simulink model "Flyback_Converter_PartA_16a"  (Simulink 8.7)
settings: Solver=ode5  SolverMode=SingleTasking  StartTime=0.0  StopTime=0.005  FixedStep=1e-7  MaxStep=1e-4  RelTol=1e-3
libraries: powerlib x14
settings Model: Creator=WINTER-SOLDIER  LastModifiedBy=nehaj
settings DataIOCC: LimitDataPoints=off  SaveFormat=Dataset
settings DebuggingCC: UnderspecifiedInitializationDetection=Simplified  MergeDetectMultiDrivingBlocksExec=error  SFUnexpectedBacktrackingDiag=error  SFNoUnconditionalDefaultTransitionDiag=error
settings HardwareCC: ProdBitPerPointer=64  ProdLargestAtomicFloat=Float  ProdIntDivRoundTo=Zero  ProdEndianess=LittleEndian  ProdWordSize=64  ProdHWDeviceType=Intel->x86-64 (Windows64)
settings ModelReferenceCC: PropagateSignalLabelsOutOfModel=on
settings GRTTargetCC: TargetLangStandard=C99 (ISO)  GeneratePreprocessorConditionals=Use local settings
settings ConfigComp: CovMetricSettings=dwe  CovHtmlReporting=off  CovSaveCumulativeToWorkspaceVar=off  CovSaveSingleToWorkspaceVar=off  CovModelRefEnable=off  CovExternalEMLEnable=on

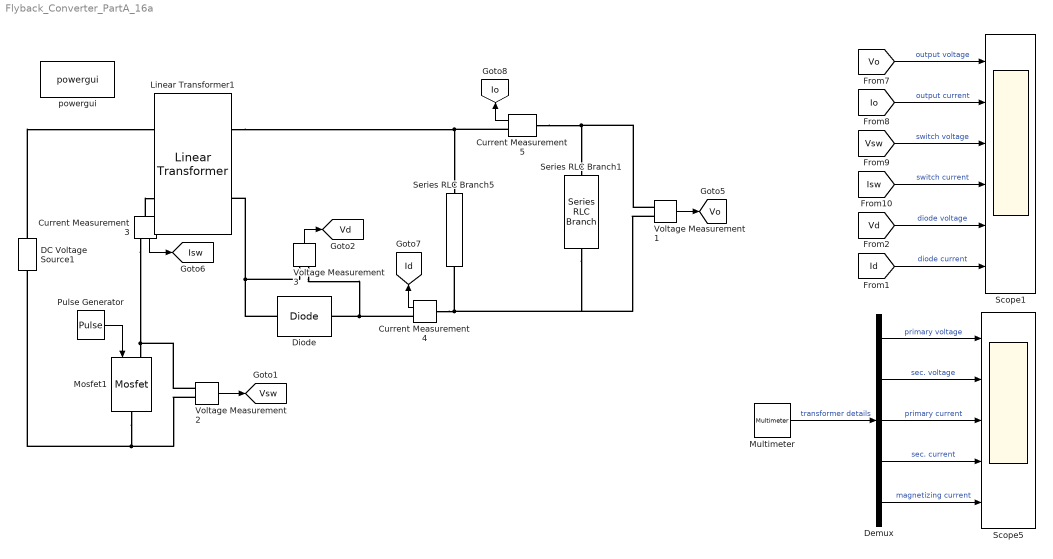
== system Flyback_Converter_PartA_16a ==
  Current Measurement3 : powerlib/Measurements/Current Measurement  PhasorSimulation=off  OutputType=Complex  PSBequivalent=0
  Current Measurement4 : powerlib/Measurements/Current Measurement  PhasorSimulation=off  OutputType=Complex  PSBequivalent=0
  Current Measurement5 : powerlib/Measurements/Current Measurement  PhasorSimulation=off  OutputType=Complex  PSBequivalent=0
  DC Voltage Source1 : powerlib/Electrical Sources/DC Voltage Source  Amplitude=20  Measurements=None
  Demux : Demux  Outputs=5
  Diode : powerlib/Power Electronics/Diode  Ron=1e-6  Lon=0  Vf=0  IC=0  UseSnubber=0  Rs=inf  Cs=0  Measurements=off
  Linear Transformer1 : powerlib/Elements/Linear Transformer  UNITS=SI  NominalPower=[20 100000 ]  winding1=[30 0 0]  winding2=[10 0 0]  ThreeWindings=off  winding3=[3.15e+05 0.7938 0.084225]  RmLm=[inf 250e-6]  Measurements=All voltages and currents  DataType=on
  Mosfet1 : powerlib/Power Electronics/Mosfet  Ron=1e-6  Lon=0  Rd=1e-6  Vfd=0  IC=0  Rs=1e12  Cs=inf  Measurements=off
  Multimeter : powerlib/Measurements/Multimeter  PhasorSimulation=off  OutputType=Complex  sel=[1 2 3 4 6]  L=7  Gain=[1 1 1 1 1]  yselected={'Uw1: Linear Transformer1','Uw2: Linear Transformer1','Iw1: Linear Transformer1','Iw2: Linear Transformer1','Imag: Linear Transformer1'};  PSBOutputType=1  PSBequivalent=0  AxesSetting=[0,0.1,-100,100]  Display=0  SavedBlockNames=-11
  Pulse Generator : DiscretePulseGenerator  PulseType=Time based  Period=1/100000  PulseWidth=50
  Scope1 : Scope  NumInputPorts=6
  Scope5 : Scope  NumInputPorts=5
  Series RLC Branch1 : powerlib/Elements/Series RLC Branch  LConnTagsString=__new0  RConnTagsString=__new0  BranchType=R  Resistance=1.5  Inductance=1e-3  SetiL0=off  InitialCurrent=0  Capacitance=1e-6  Setx0=off  InitialVoltage=0  Measurements=None
  Series RLC Branch5 : powerlib/Elements/Series RLC Branch  LConnTagsString=__new0  RConnTagsString=__new0  BranchType=C  Resistance=0  Inductance=1e-3  SetiL0=off  InitialCurrent=0  Capacitance=100e-6  Setx0=off  InitialVoltage=0  Measurements=None
  Voltage Measurement1 : powerlib/Measurements/Voltage Measurement  PhasorSimulation=off  OutputType=Complex  PSBequivalent=0
  Voltage Measurement2 : powerlib/Measurements/Voltage Measurement  PhasorSimulation=off  OutputType=Complex  PSBequivalent=0
  Voltage Measurement3 : powerlib/Measurements/Voltage Measurement  PhasorSimulation=off  OutputType=Complex  PSBequivalent=0
  powergui : powerlib/powergui  Priority=1  SimulationMode=Discrete  SampleTime=1e-7  frequency=60  Iterations=50  frequencyindice=0  Pbase=100e6  ErrMax=1e-4  UnitsV=kV  UnitsW=MW  buscounter=0  FunctionMessages=off  echomessages=off  EnableUseOfTLC=off  CurrentSourceSwitches=off  DisableSnubberDevices=off  DisableRonSwitches=off  DisableVfSwitches=off  DisplayEquations=off  SolverType=Tustin/Backward Euler (TBE)  Interpol=off  ExternalGateDelay=off  methode=off  Ts=100  x0status=blocks  SPID=on  SwTol=0  HookPort=off  RestoreLinks=warning  ResistiveCurrentMeasurement=off  Frange=[0:2:500]  Ylog=off  Xlog=on  ShowGrid=off  save=off  variable=ZData  structure=0  ZoomFFT=off  StartTime=0.0  cycles=1  DisplayStyle=1  fundamental=60  FreqAxis=off  MaxFrequency=1000  frequencyindicesteady=1  RmsSteady=1  display=off
  tag scope: Id=global, Io=global, Isw=global, Vd=global, Vo=global, Vsw=global
  wires:
  Voltage Measurement1/1 -> [Vo]
  Pulse Generator/1 -> Mosfet1/1
  Current Measurement5/1 -> [Io]
  Current Measurement3/1 -> [Isw]
  Current Measurement4/1 -> [Id]
  [Vsw] -> Scope1/3  "switch voltage"
  [Vo] -> Scope1/1  "output voltage"
  [Io] -> Scope1/2  "output current"
  [Isw] -> Scope1/4  "switch current"
  Voltage Measurement2/1 -> [Vsw]
  [Vd] -> Scope1/5  "diode voltage"
  [Id] -> Scope1/6  "diode current"
  Voltage Measurement3/1 -> [Vd]
  Demux/1 -> Scope5/1  "primary voltage"
  Multimeter/1 -> Demux/1  "transformer details"
  Demux/2 -> Scope5/2  "sec. voltage"
  Demux/5 -> Scope5/5  "magnetizing current"
  Demux/3 -> Scope5/3  "primary current"
  Demux/4 -> Scope5/4  "sec. current"
  connections:
  Linear Transformer1/RConn1 -- Series RLC Branch5/RConn1 -- Current Measurement5/RConn1
  Mosfet1/RConn1 -- DC Voltage Source1/LConn1 -- Voltage Measurement2/LConn2
  DC Voltage Source1/RConn1 -- Linear Transformer1/LConn1
  Current Measurement3/RConn1 -- Voltage Measurement2/LConn1 -- Mosfet1/LConn1
  Current Measurement3/LConn1 -- Linear Transformer1/LConn2
  Current Measurement4/RConn1 -- Diode/RConn1 -- Voltage Measurement3/LConn2
  Diode/LConn1 -- Voltage Measurement3/LConn1 -- Linear Transformer1/RConn2
  Current Measurement4/LConn1 -- Voltage Measurement1/LConn1 -- Series RLC Branch1/LConn1 -- Series RLC Branch5/LConn1
  Voltage Measurement1/LConn2 -- Current Measurement5/LConn1 -- Series RLC Branch1/RConn1
